simulink model "mlp_mid_level_processor_hrn"  (R2015a)
settings: Solver=ode3  StartTime=0.0  StopTime=mlp_stop_time  FixedStep=astrobee_time_step_size  RelTol=1e-3
undefined symbols (not defined in the file or in its folder): astrobee_time_step_size
libraries: util_test_utilities_lib x1, mlp_mid_level_processor_lib x1, env_environment_model_lib x1
settings Model: Creator=rhnakamu  LastModifiedBy=rhnakamu

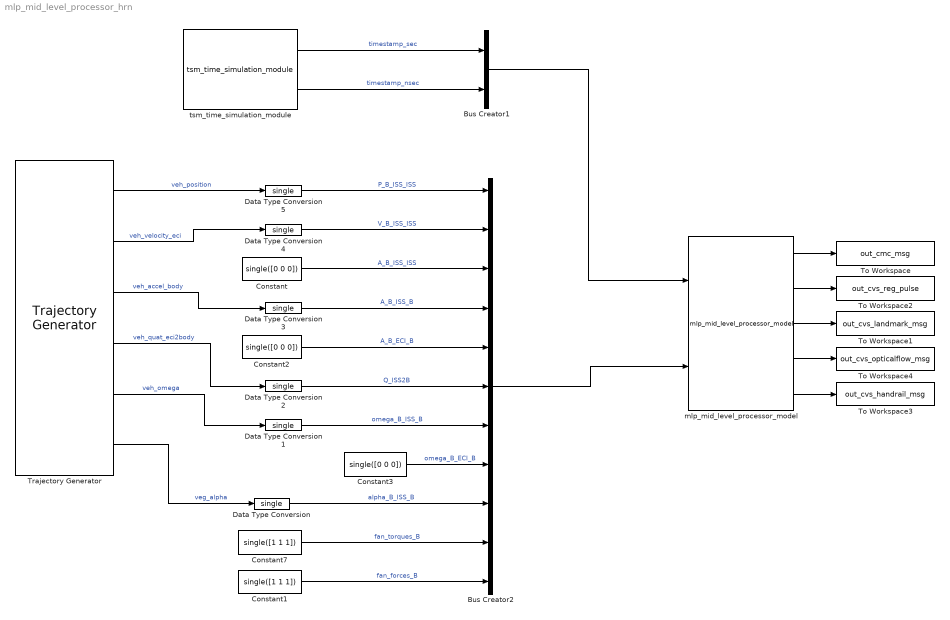
== system mlp_mid_level_processor_hrn ==
  Bus Creator1 : BusCreator  Inputs=2  OutDataTypeStr=Bus: ex_time_msg  NonVirtualBus=on
      settings: InheritFromInputs=off
  Bus Creator2 : BusCreator  Inputs=11  OutDataTypeStr=Bus: env_msg  NonVirtualBus=on
      settings: InheritFromInputs=off
  Constant : Constant  Value=single([0 0 0])
  Constant1 : Constant  Value=single([1 1 1])
  Constant2 : Constant  Value=single([0 0 0])
  Constant3 : Constant  Value=single([0 0 0])
  Constant7 : Constant  Value=single([1 1 1])
  Data Type Conversion{,1..5} (6 alike) : DataTypeConversion  OutDataTypeStr=single
  To Workspace : ToWorkspace  VariableName=out_cmc_msg  SaveFormat=Timeseries  SampleTime=-1
  To Workspace1 : ToWorkspace  VariableName=out_cvs_landmark_msg  SaveFormat=Timeseries  SampleTime=-1
  To Workspace2 : ToWorkspace  VariableName=out_cvs_reg_pulse  SaveFormat=Timeseries  SampleTime=-1
  To Workspace3 : ToWorkspace  VariableName=out_cvs_handrail_msg  SaveFormat=Timeseries  SampleTime=-1
  To Workspace4 : ToWorkspace  VariableName=out_cvs_opticalflow_msg  SaveFormat=Timeseries  SampleTime=-1
  Trajectory Generator : util_test_utilities_lib/Trajectory Generator  wpoints=wpts_lin  time_pts=wpts_t_lin  omega_vec=wpts_ang  omega_time=wpts_t_ang  quat_init=[0, 0, 0, 1]  Ts=astrobee_time_step_size
  mlp_mid_level_processor_model : mlp_mid_level_processor_lib/mlp_mid_level_processor_model
  tsm_time_simulation_module : env_environment_model_lib/env_environment_model/tsm_time_simulation_module
  wires:
  Constant1/1 -> Bus Creator2/11  "fan_forces_B"
  Constant7/1 -> Bus Creator2/10  "fan_torques_B"
  mlp_mid_level_processor_model/3 -> To Workspace1/1
  mlp_mid_level_processor_model/1 -> To Workspace/1
  mlp_mid_level_processor_model/2 -> To Workspace2/1
  mlp_mid_level_processor_model/4 -> To Workspace4/1
  Trajectory Generator/2 -> Data Type Conversion4/1  "veh_velocity_eci"
  Trajectory Generator/1 -> Data Type Conversion5/1  "veh_position"
  Bus Creator2/1 -> mlp_mid_level_processor_model/2
  Bus Creator1/1 -> mlp_mid_level_processor_model/1
  Constant/1 -> Bus Creator2/3  "A_B_ISS_ISS"
  Trajectory Generator/6 -> Data Type Conversion/1  "veg_alpha"
  Trajectory Generator/5 -> Data Type Conversion1/1  "veh_omega"
  Trajectory Generator/4 -> Data Type Conversion2/1  "veh_quat_eci2body"
  Trajectory Generator/3 -> Data Type Conversion3/1  "veh_accel_body"
  tsm_time_simulation_module/2 -> Bus Creator1/2  "timestamp_nsec"
  tsm_time_simulation_module/1 -> Bus Creator1/1  "timestamp_sec"
  Data Type Conversion/1 -> Bus Creator2/9  "alpha_B_ISS_B"
  Data Type Conversion1/1 -> Bus Creator2/7  "omega_B_ISS_B"
  Data Type Conversion2/1 -> Bus Creator2/6  "Q_ISS2B"
  Data Type Conversion3/1 -> Bus Creator2/4  "A_B_ISS_B"
  Data Type Conversion4/1 -> Bus Creator2/2  "V_B_ISS_ISS"
  Data Type Conversion5/1 -> Bus Creator2/1  "P_B_ISS_ISS"
  Constant2/1 -> Bus Creator2/5  "A_B_ECI_B"
  Constant3/1 -> Bus Creator2/8  "omega_B_ECI_B"
  mlp_mid_level_processor_model/5 -> To Workspace3/1
